simulink model "MRAC_indireto_111_8_5"  (Simulink 8.5)
settings: Solver=ode45  SolverMode=SingleTasking  StartTime=0.0  StopTime=40.0  RelTol=1e-3  AbsTol=1e-6
values from neighbouring files (symbols this model uses):
  af = 1    [parameters.m]    (also in simu_gradiente.m = 0.5; simu_indireto.m)
  am = 1    [parameters.m]    (also in simu01.m; simu02.m; simu03.m; simu04.m)
  As = 0    [parameters.m]    (also in simu01.m; simu02.m; simu03.m; simu04.m)
  DC = 1    [parameters.m]    (also in simu01.m; simu02.m; simu03.m; simu04.m)
  gamma = 10    [parameters.m]    (also in simu01.m = 100; simu02.m = 100; simu03.m = 100; simu04.m)
  m_type = 2    [simu02.m]    (also in simu_gradiente.m; simu_indireto.m)
  st = 0.05    [parameters.m]    (also in simu01.m; simu02.m; simu03.m = 0.001; simu04.m)
  theta0 = 0    [parameters.m]    (also in simu01.m; simu02.m; simu03.m; simu04.m)
  ws = 10    [parameters.m]    (also in simu01.m; simu02.m; simu03.m = 1; simu04.m)
libraries: cstblocks x2
settings Model: Creator=Ramon  LastModifiedBy=renan
settings DataIOCC: LimitDataPoints=off  SaveOutput=off  SaveTime=off
settings OptimizationCC: BlockReduction=off  BooleanDataType=off  InitFltsAndDblsToZero=on
settings DebuggingCC: SaveWithParameterizedLinksMsg=none  SignalResolutionControl=TryResolveAllWithWarning  MultiTaskDSMMsg=warning  MultiTaskCondExecSysMsg=none  FcnCallInpInsideContextMsg=EnableAllAsWarning
settings HardwareCC: TargetUnknown=on
settings RTWCC: TemplateMakefile=grt_vc.tmf

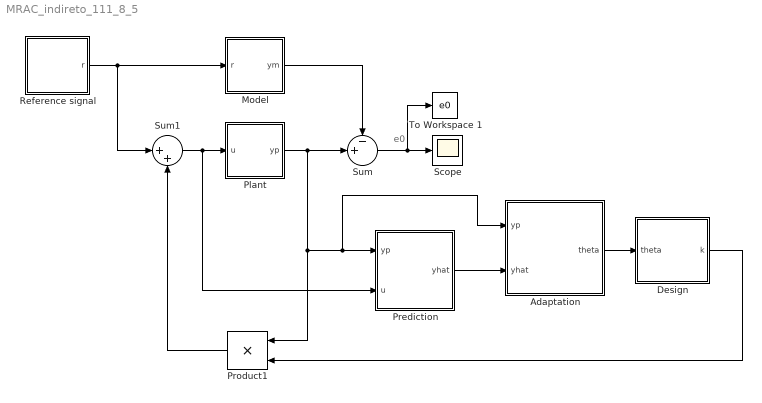
== system MRAC_indireto_111_8_5 ==
  note: e0
  Adaptation : Subsystem
  Design : Subsystem
  Model : Subsystem
  Plant : Subsystem
  Prediction : Subsystem
  Product1 : Product  SaturateOnIntegerOverflow=on  RndMeth=Zero  InputSameDT=on  OutDataTypeStr=Inherit: Same as first input
  Reference signal : Subsystem
  Scope : Scope
      settings: TimeRange=20  TickLabels=on  LimitDataPoints=on  MaxDataPoints=5000  SaveToWorkspace=off  SaveName=ScopeData  YMin=-1  YMax=2  SampleTime=-1  DataFormat=Array
  Sum : Sum  Inputs=-+|  SaturateOnIntegerOverflow=on  InputSameDT=on  OutDataTypeStr=Inherit: Same as first input
  Sum1 : Sum  Inputs=|++  SaturateOnIntegerOverflow=on  InputSameDT=on  OutDataTypeStr=Inherit: Same as first input
  To Workspace 1 : ToWorkspace  VariableName=e0  SampleTime=st
  wires:
  Sum/1 -> Scope/1, To Workspace 1/1
  Model/1(ym) -> Sum/1
  Plant/1(yp) -> Sum/2, Adaptation/1(yp), Prediction/1(yp), Product1/1
  Reference signal/1(r) -> Model/1(r), Sum1/1
  Sum1/1 -> Plant/1(u), Prediction/2(u)
  Product1/1 -> Sum1/2
  Adaptation/1(theta) -> Design/1(theta)
  Design/1(k) -> Product1/2
  Prediction/1(yhat) -> Adaptation/2(yhat)

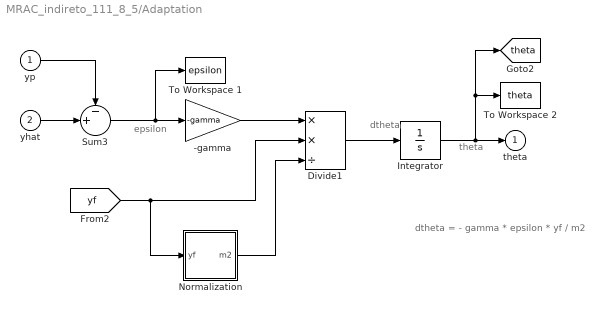
== system MRAC_indireto_111_8_5/Adaptation ==
  note: theta
  note: dtheta
  note: epsilon
  note: dtheta = - gamma * epsilon * yf / m2
  yp : Inport  PortDimensions=1
  yhat : Inport  Port=2
  -gamma : Gain  Gain=-gamma  SaturateOnIntegerOverflow=on  OutDataTypeStr=Inherit: Same as input  ParamDataTypeStr=Inherit: Same as input
  Divide1 : Product  Inputs=**/
  Integrator : Integrator  InitialCondition=theta0
  Normalization : Subsystem
  Sum3 : Sum  Inputs=-+|  SaturateOnIntegerOverflow=on  InputSameDT=on  OutDataTypeStr=Inherit: Same as first input
  To Workspace 1 : ToWorkspace  VariableName=epsilon  SampleTime=st
  To Workspace 2 : ToWorkspace  VariableName=theta  SampleTime=st
  theta : Outport  InitialOutput=0
  tag scope: theta=global
  wires:
  Divide1/1 -> Integrator/1
  Integrator/1 -> To Workspace 2/1, [theta], theta/1
  yp/1 -> Sum3/1
  Sum3/1 -> -gamma/1, To Workspace 1/1
  yhat/1 -> Sum3/2
  -gamma/1 -> Divide1/1
  Normalization/1(m2) -> Divide1/3
  [yf] -> Divide1/2, Normalization/1(yf)

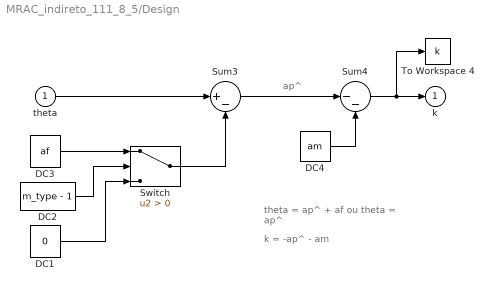
== system MRAC_indireto_111_8_5/Design ==
  note: ap^
  note: theta = ap^ + af ou theta = ap^
  note: k = -ap^ - am
  theta : Inport  PortDimensions=1
  DC1 : Constant  Value=0
  DC2 : Constant  Value=m_type - 1
  DC3 : Constant  Value=af
  DC4 : Constant  Value=am
  Sum3 : Sum  Inputs=|+-  SaturateOnIntegerOverflow=on  InputSameDT=on  OutDataTypeStr=Inherit: Same as first input
  Sum4 : Sum  Inputs=|--  SaturateOnIntegerOverflow=on  InputSameDT=on  OutDataTypeStr=Inherit: Same as first input
  Switch : Switch  Criteria=u2 > Threshold
  To Workspace 4 : ToWorkspace  VariableName=k  SampleTime=st
  k : Outport  InitialOutput=0
  wires:
  Sum4/1 -> To Workspace 4/1, k/1
  theta/1 -> Sum3/1
  Sum3/1 -> Sum4/1
  DC4/1 -> Sum4/2
  DC2/1 -> Switch/2
  DC1/1 -> Switch/3
  DC3/1 -> Switch/1
  Switch/1 -> Sum3/2

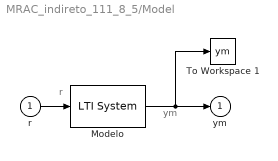
== system MRAC_indireto_111_8_5/Model ==
  note: r
  note: ym
  r : Inport
  Modelo : cstblocks/LTI System  sys=M  IC=ym0
  To Workspace 1 : ToWorkspace  VariableName=ym  SampleTime=st
  ym : Outport  InitialOutput=0
  wires:
  Modelo/1 -> To Workspace 1/1, ym/1
  r/1 -> Modelo/1

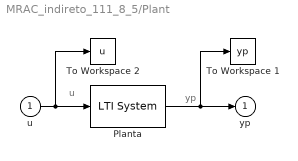
== system MRAC_indireto_111_8_5/Plant ==
  note: yp
  note: u
  u : Inport
  Planta : cstblocks/LTI System  sys=P  IC=yp0
  To Workspace 1 : ToWorkspace  VariableName=yp  SampleTime=st
  To Workspace 2 : ToWorkspace  VariableName=u  SampleTime=st
  yp : Outport  InitialOutput=0
  wires:
  u/1 -> To Workspace 2/1, Planta/1
  Planta/1 -> yp/1, To Workspace 1/1

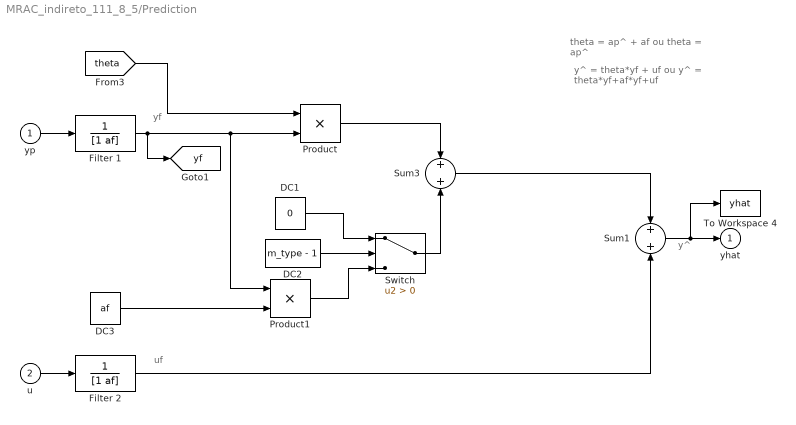
== system MRAC_indireto_111_8_5/Prediction ==
  note: yf
  note: uf
  note: y^ = theta*yf + uf ou y^ = theta*yf+af*yf+uf
  note: theta = ap^ + af ou theta = ap^
  note: y^
  yp : Inport
  u : Inport  Port=2
  DC1 : Constant  Value=0
  DC2 : Constant  Value=m_type - 1
  DC3 : Constant  Value=af
  Filter 1 : TransferFcn  Denominator=[1 af]
  Filter 2 : TransferFcn  Denominator=[1 af]
  Product : Product  SaturateOnIntegerOverflow=on  RndMeth=Zero  InputSameDT=on  OutDataTypeStr=Inherit: Same as first input
  Product1 : Product  SaturateOnIntegerOverflow=on  RndMeth=Zero  InputSameDT=on  OutDataTypeStr=Inherit: Same as first input
  Sum1 : Sum  Inputs=+|+  SaturateOnIntegerOverflow=on  InputSameDT=on  OutDataTypeStr=Inherit: Same as first input
  Sum3 : Sum  Inputs=+|+  SaturateOnIntegerOverflow=on  InputSameDT=on  OutDataTypeStr=Inherit: Same as first input
  Switch : Switch  Criteria=u2 > Threshold
  To Workspace 4 : ToWorkspace  VariableName=yhat  SampleTime=st
  yhat : Outport  InitialOutput=0
  tag scope: yf=global
  wires:
  yp/1 -> Filter 1/1
  u/1 -> Filter 2/1
  [theta] -> Product/1
  Product/1 -> Sum3/1
  Sum1/1 -> yhat/1, To Workspace 4/1
  Filter 2/1 -> Sum1/2
  Filter 1/1 -> Product/2, Product1/1, [yf]
  DC3/1 -> Product1/2
  Sum3/1 -> Sum1/1
  Switch/1 -> Sum3/2
  DC2/1 -> Switch/2
  DC1/1 -> Switch/1
  Product1/1 -> Switch/3

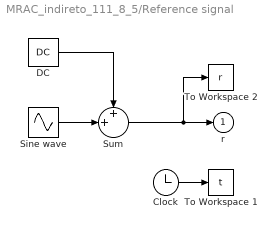
== system MRAC_indireto_111_8_5/Reference signal ==
  Clock : Clock
  DC : Constant  Value=DC
  Sine wave : Sin  Amplitude=As  Frequency=ws  SampleTime=0
  Sum : Sum  Inputs=++|  SaturateOnIntegerOverflow=on  InputSameDT=on  OutDataTypeStr=Inherit: Same as first input
  To Workspace 1 : ToWorkspace  VariableName=t  SampleTime=st
  To Workspace 2 : ToWorkspace  VariableName=r  SampleTime=st
  r : Outport  InitialOutput=0
  wires:
  DC/1 -> Sum/1
  Sum/1 -> r/1, To Workspace 2/1
  Clock/1 -> To Workspace 1/1
  Sine wave/1 -> Sum/2

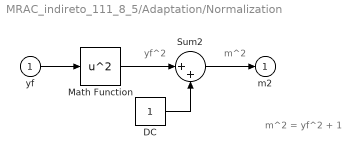
== system MRAC_indireto_111_8_5/Adaptation/Normalization ==
  note: yf^2
  note: m^2
  note: m^2 = yf^2 + 1
  yf : Inport  PortDimensions=1
  DC : Constant
  Math Function : Math  Operator=square  SaturateOnIntegerOverflow=on
  Sum2 : Sum  Inputs=|++  SaturateOnIntegerOverflow=on  InputSameDT=on  OutDataTypeStr=Inherit: Same as first input
  m2 : Outport  InitialOutput=0
  wires:
  yf/1 -> Math Function/1
  Math Function/1 -> Sum2/1
  DC/1 -> Sum2/2
  Sum2/1 -> m2/1
